simulink model "button_to_pulse"  (R2014a)
settings: Solver=ode45  StartTime=0.0  StopTime=50000  RelTol=1e-3
libraries: hdlsllib x4, simulink x2
settings Model: Creator=scherb.a  LastModifiedBy=scherb.a

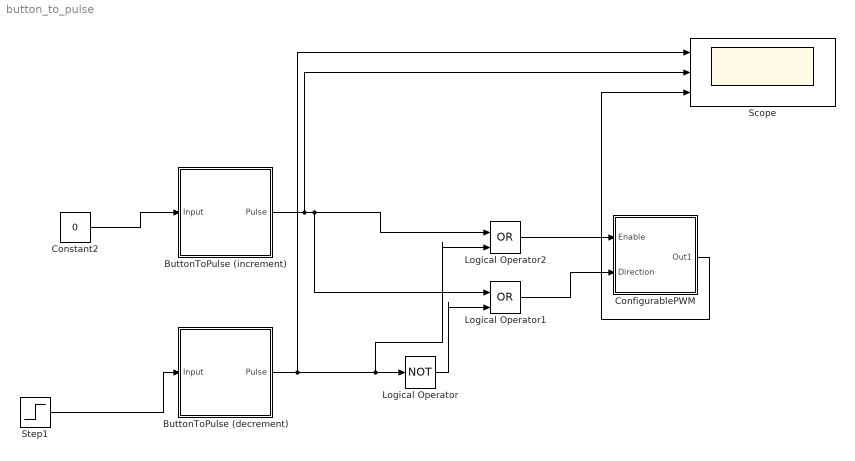
== system button_to_pulse ==
  ButtonToPulse (decrement) : Subsystem
  ButtonToPulse (increment) : Subsystem
  ConfigurablePWM : Subsystem
  Constant2 : Constant  Value=0
  Logical Operator : Logic  Operator=NOT  IconShape=distinctive  AllPortsSameDT=off  OutDataTypeStr=boolean
  Logical Operator1 : Logic  Operator=OR  IconShape=distinctive  AllPortsSameDT=off  OutDataTypeStr=boolean
  Logical Operator2 : Logic  Operator=OR  IconShape=distinctive  AllPortsSameDT=off  OutDataTypeStr=boolean
  Scope : Scope  NumInputPorts=3
      settings: YMin=-5~-5~-5  YMax=5~5~5
  Step1 : Step  Time=25000  Before=1  After=0  SampleTime=50000
  wires:
  Logical Operator2/1 -> ConfigurablePWM/1(Enable)
  Logical Operator1/1 -> ConfigurablePWM/2(Direction)
  Logical Operator/1 -> Logical Operator1/2
  ButtonToPulse (decrement)/1(Pulse) -> Scope/1, Logical Operator2/2, Logical Operator/1
  ButtonToPulse (increment)/1(Pulse) -> Scope/2, Logical Operator1/1, Logical Operator2/1
  ConfigurablePWM/1(Out1) -> Scope/3
  Step1/1 -> ButtonToPulse (decrement)/1(Input)
  Constant2/1 -> ButtonToPulse (increment)/1(Input)

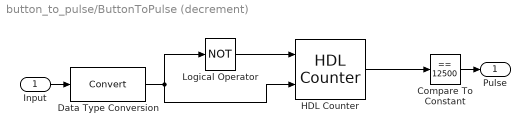
== system button_to_pulse/ButtonToPulse (decrement) ==
  Input : Inport
  Compare To Constant : simulink/Logic and Bit Operations/Compare To Constant  relop===  const=12500  OutDataTypeStr=boolean
  Data Type Conversion : DataTypeConversion
  HDL Counter : hdlsllib/HDL Operations/HDL Counter  CountType=Count limited  CountInit=0  CountStep=1  CountMax=50000  CountFromType=Initial value  CountFrom=0  CountResetPort=on  CountLoadPort=off  CountEnbPort=on  CountDirPort=off  CountDataType=Unsigned  CountWordLen=32  CountFracLen=0  CountSampTime=1
  Logical Operator : Logic  Operator=NOT  IconShape=distinctive  AllPortsSameDT=off  OutDataTypeStr=boolean
  Pulse : Outport
  wires:
  HDL Counter/1 -> Compare To Constant/1
  Logical Operator/1 -> HDL Counter/1
  Data Type Conversion/1 -> HDL Counter/2, Logical Operator/1
  Compare To Constant/1 -> Pulse/1
  Input/1 -> Data Type Conversion/1

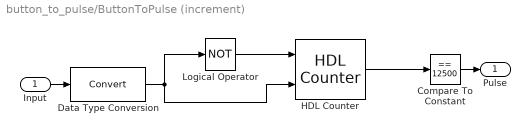
== system button_to_pulse/ButtonToPulse (increment) ==
  Input : Inport
  Compare To Constant : simulink/Logic and Bit Operations/Compare To Constant  relop===  const=12500  OutDataTypeStr=boolean
  Data Type Conversion : DataTypeConversion
  HDL Counter : hdlsllib/HDL Operations/HDL Counter  CountType=Count limited  CountInit=0  CountStep=1  CountMax=50000  CountFromType=Initial value  CountFrom=0  CountResetPort=on  CountLoadPort=off  CountEnbPort=on  CountDirPort=off  CountDataType=Unsigned  CountWordLen=32  CountFracLen=0  CountSampTime=1
  Logical Operator : Logic  Operator=NOT  IconShape=distinctive  AllPortsSameDT=off  OutDataTypeStr=boolean
  Pulse : Outport
  wires:
  HDL Counter/1 -> Compare To Constant/1
  Logical Operator/1 -> HDL Counter/1
  Data Type Conversion/1 -> HDL Counter/2, Logical Operator/1
  Compare To Constant/1 -> Pulse/1
  Input/1 -> Data Type Conversion/1

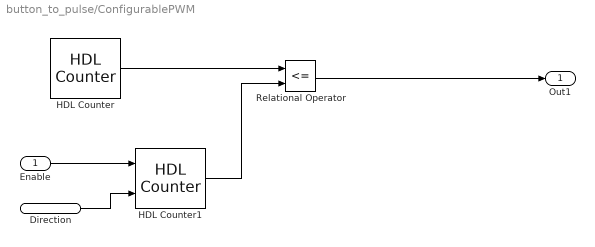
== system button_to_pulse/ConfigurablePWM ==
  Enable : Inport
  Direction : Inport  Port=2
  HDL Counter : hdlsllib/HDL Operations/HDL Counter  CountType=Count limited  CountInit=0  CountStep=1  CountMax=1000  CountFromType=Initial value  CountFrom=0  CountResetPort=off  CountLoadPort=off  CountEnbPort=off  CountDirPort=off  CountDataType=Unsigned  CountWordLen=20  CountFracLen=0  CountSampTime=1
  HDL Counter1 : hdlsllib/HDL Operations/HDL Counter  CountType=Count limited  CountInit=75  CountStep=6  CountMax=120  CountFromType=Specify  CountFrom=30  CountResetPort=off  CountLoadPort=off  CountEnbPort=on  CountDirPort=on  CountDataType=Unsigned  CountWordLen=8  CountFracLen=0  CountSampTime=1
  Relational Operator : RelationalOperator  Operator=<=  OutDataTypeStr=boolean
  Out1 : Outport
  wires:
  Enable/1 -> HDL Counter1/1
  HDL Counter1/1 -> Relational Operator/2
  Direction/1 -> HDL Counter1/2
  HDL Counter/1 -> Relational Operator/1
  Relational Operator/1 -> Out1/1
